simulink model "Simulink_Offline_Horizontal_Control"  (R2022b)
settings: Solver=VariableStepAuto  StartTime=0.0  StopTime=10.0  RelTol=1e-3
values from neighbouring files (symbols this model uses):
  C = eye(4)    [PID_tuner.m]
  D = zeros(4,1)    [PID_tuner.m]
  Kd = G.Kd    [PID_tuner.m]
  Ki = G.Ki    [PID_tuner.m]
  Kp = G.Kp    [PID_tuner.m]
undefined symbols (not defined in the file or in its folder): A, B
libraries: slpidlib x1
settings Model: Creator=utente  LastModifiedBy=albif
settings SolverCC: AlgebraicLoopSolver=TrustRegion
settings DebuggingCC: UnconnectedInputMsg=warning  UnconnectedOutputMsg=warning  UnconnectedLineMsg=warning  SFMachineParentedDataDiag=warning
settings ModelReferenceCC: EnableRefExpFcnMdlSchedulingChecks=on

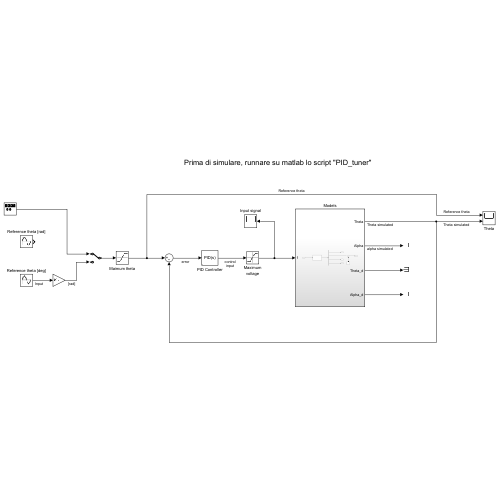
[thumbnail: Simulink's stored preview of the top-level diagram]
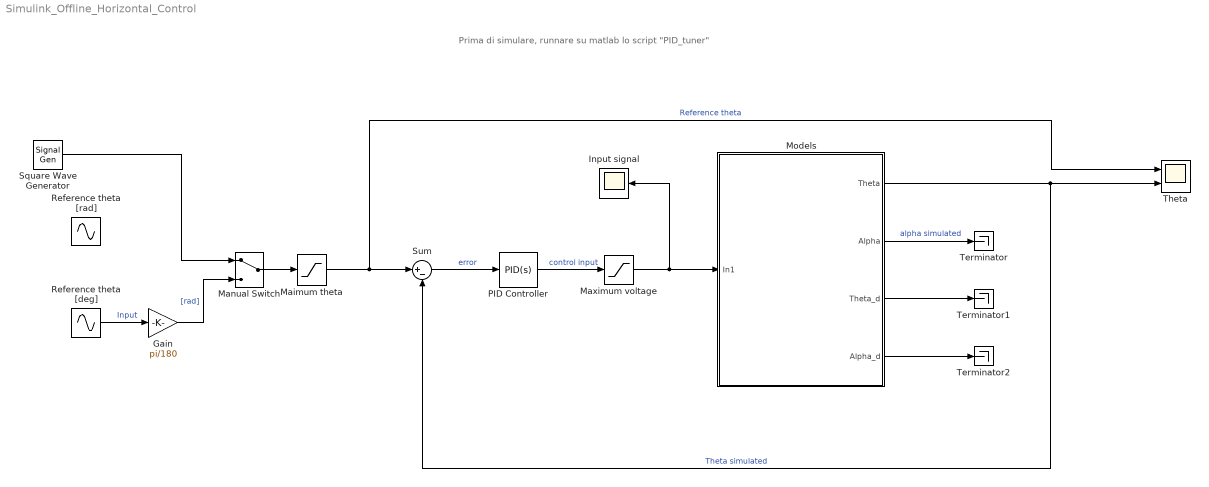
== system Simulink_Offline_Horizontal_Control ==
  note: Prima di simulare, runnare su matlab lo script "PID_tuner"
  Gain : Gain  Gain=pi/180
  Input signal : Scope
  Maimum theta : Saturate  UpperLimit=pi/2  LowerLimit=-pi/2
  Manual Switch : ManualSwitch
  Maximum voltage : Saturate  UpperLimit=6  LowerLimit=-6
  Models : Subsystem
  PID Controller : slpidlib/PID Controller  Controller=PID  Form=Parallel  TimeDomain=Continuous-time  UseExternalTs=off  SampleTime=-1  IntegratorMethod=Forward Euler  FilterMethod=Forward Euler  ControllerParametersSource=internal  P=Kp  I=Ki  UseKiTs=off  D=Kd  N=10  UseFilter=on  TunerSelectOption=Transfer Function Based (PID Tuner App)  InitialConditionSource=internal  InitialConditionForIntegrator=0  InitialConditionForFilter=0  DifferentiatorICPrevScaledInput=0  ExternalReset=none  TrackingMode=off  Kt=1  LimitOutput=off  SatLimitsSource=internal  UpperSaturationLimit=inf  LowerSaturationLimit=-inf  LinearizeAsGain=on  AntiWindupMode=none  Kb=1  LimitIntegrator=off  UpperIntegratorSaturationLimit=inf  LowerIntegratorSaturationLimit=-inf  POutMin=[]  POutMax=[]  IOutMin=[]  IOutMax=[]  DOutMin=[]  DOutMax=[]  NOutMin=[]  NOutMax=[]  SumOutMin=[]  SumOutMax=[]  SaturationOutMin=[]  SaturationOutMax=[]  PParamMin=[]  PParamMax=[]  IParamMin=[]  IParamMax=[]  DParamMin=[]  DParamMax=[]  NParamMin=[]  NParamMax=[]  KbParamMin=[]  KbParamMax=[]  KtParamMin=[]  KtParamMax=[]  KbOutMin=[]  KbOutMax=[]  KtOutMin=[]  KtOutMax=[]  IntegratorOutMin=[]  IntegratorOutMax=[]  FilterOutMin=[]  FilterOutMax=[]  SumI1OutMin=[]  SumI1OutMax=[]  SumI2OutMin=[]  SumI2OutMax=[]  SumI3OutMin=[]  SumI3OutMax=[]  SumI4OutMin=[]  SumI4OutMax=[]  SumDOutMin=[]  SumDOutMax=[]  DifferentiatorOutMin=[]  DifferentiatorOutMax=[]  FilterDiffOutCoefMin=[]  FilterDiffOutCoefMax=[]  ReciprocalOutMin=[]  ReciprocalOutMax=[]  SumDenOutMin=[]  SumDenOutMax=[]  SumNumOutMin=[]  SumNumOutMax=[]  DivideOutMin=[]  DivideOutMax=[]  UdiffTsProdOutMin=[]  UdiffTsProdOutMax=[]  NTsProdOutMin=[]  NTsProdOutMax=[]  UintegralTsProdOutMin=[]  UintegralTsProdOutMax=[]  UngainTsProdOutMin=[]  UngainTsProdOutMax=[]  ClampingZeroOutDataTypeStr=Inherit: Inherit via back propagation  ClampingZeroOutMin=[]  ClampingZeroOutMax=[]  FilterDenConstantOutDataTypeStr=Inherit: Inherit via back propagation  FilterDenConstantOutMin=[]  FilterDenConstantOutMax=[]  PCopyOutDataTypeStr=Inherit: Inherit via back propagation  PCopyOutMin=[]  PCopyOutMax=[]  NCopyOutDataTypeStr=Inherit: Inherit via back propagation  NCopyOutMin=[]  NCopyOutMax=[]  IntegratorContinuousStateAttributes=''  IntegratorStateMustResolveToSignalObject=off  IntegratorRTWStateStorageClass=Auto  FilterContinuousStateAttributes=''  FilterStateMustResolveToSignalObject=off  FilterRTWStateStorageClass=Auto  ParallelPVariant=InternalParameters  IdealPVariant=Disabled  IVariant=InternalParameters  DVariant=InternalParameters  IntegratorVariant=Continuous  SatVariant=Disabled  AWVariant=Passthrough  PCopyVariant=Disabled  TRVariant=Disabled  FdbkBlocksVariant=Forward  IdealPFdbkVariant=Disabled  SatFdbkVariant=Disabled  DerivativeFilterVariant=ContFilter  NVariant=InternalParameters  NCopyVariant=Disabled  FilterICVariant=InternalICsFilter  IntegratorICVariant=InternalICs  ExternalResetVariant=Disabled  TRSumVariant=Passthrough  SumFdbkVariant=Disabled  SumVariant=Sum_PID  TsampFilterVariant=InternalTs  TsampNgainVariant=Passthrough  TsampIntegralVariant=Passthrough  ExternalSaturationOutDataTypeStr=Inherit: Same as second input
  Reference theta [deg] : Sin  Amplitude=45  SampleTime=0
  Reference theta [rad] : Sin  Amplitude=pi/4  SampleTime=0
  Square Wave Generator : SignalGenerator  WaveForm=square  Amplitude=pi/4  Frequency=0.1
  Sum : Sum  Inputs=|+-
  Terminator : Terminator
  Terminator1 : Terminator
  Terminator2 : Terminator
  Theta : Scope  NumInputPorts=2
  wires:
  Models/1(Theta) -> Theta/2, Sum/2  "Theta simulated"
  Models/2(Alpha) -> Terminator/1  "alpha simulated"
  Models/3(Theta_d) -> Terminator1/1
  Models/4(Alpha_d) -> Terminator2/1
  Manual Switch/1 -> Maimum theta/1
  Maximum voltage/1 -> Models/1(In1), Input signal/1
  Sum/1 -> PID Controller/1  "error"
  PID Controller/1 -> Maximum voltage/1  "control input"
  Maimum theta/1 -> Sum/1, Theta/1  "Reference theta"
  Gain/1 -> Manual Switch/2  "[rad]"
  Reference theta [deg]/1 -> Gain/1  "Input"
  Square Wave Generator/1 -> Manual Switch/1

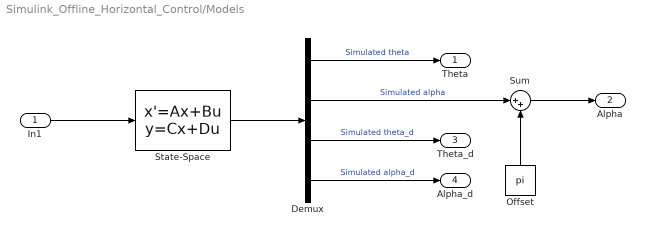
== system Simulink_Offline_Horizontal_Control/Models ==
  In1 : Inport
  Demux : Demux
  Offset : Constant  Value=pi
  State-Space : StateSpace  A=A  B=B  C=C  D=D  InitialCondition=0
  Sum : Sum  Inputs=|++
  Theta : Outport
  Alpha : Outport  Port=2
  Theta_d : Outport  Port=3
  Alpha_d : Outport  Port=4
  wires:
  In1/1 -> State-Space/1
  Demux/1 -> Theta/1  "Simulated theta"
  Demux/2 -> Sum/1  "Simulated alpha"
  State-Space/1 -> Demux/1
  Demux/4 -> Alpha_d/1  "Simulated alpha_d"
  Demux/3 -> Theta_d/1  "Simulated theta_d"
  Sum/1 -> Alpha/1
  Offset/1 -> Sum/2
